simulink model "VisionModel_v8"  (Simulink 7.6)
settings: Solver=FixedStepDiscrete  StartTime=0.0  StopTime=0  RelTol=1e-3
values from neighbouring files (symbols this model uses):
  Buoy_Max_Eccentricity = 1.2    [VisionConstants.m]
  Buoy_Max_Extent = 0.9    [VisionConstants.m]
  Buoy_Min_Eccentricity = 0    [VisionConstants.m]
  Buoy_Min_Extent = 0.1    [VisionConstants.m]
  Forward_Camera_Dimensions = [160 120]    [VisionConstants.m]
  Iter_Segment_Thresh = 60    [VisionConstants.m]
  Scale_Down_B = 1    [VisionConstants.m]
  Scale_Down_G = 1    [VisionConstants.m]
  Scale_Down_H = 1    [VisionConstants.m]
  Scale_Down_R = 1    [VisionConstants.m]
  Scale_Down_S = 1    [VisionConstants.m]
  Scale_Down_V = 5    [VisionConstants.m]
  Scale_Forward_B = 0    [VisionConstants.m]
  Scale_Forward_G = 1    [VisionConstants.m]
  Scale_Forward_H = 1    [VisionConstants.m]
  Scale_Forward_R = 0    [VisionConstants.m]
  Scale_Forward_S = 1    [VisionConstants.m]
  Scale_Forward_V = 5    [VisionConstants.m]
undefined symbols (not defined in the file or in its folder): Forward_Fov, Rec, SDTV
libraries: vipconversions x8, vipgeotforms x6, viptextngfix x4, vipanalysis x2, viptransforms x2
(part 1 of 3)
settings Model: Creator=Administrator  LastModifiedBy=auvt
settings OptimizationCC: OptimizeModelRefInitCode=on
settings RTWCC: SystemTargetFile=ert.tlc  GenCodeOnly=on  TemplateMakefile=ert_default_tmf  PostCodeGenCommand=packNGo(buildInfo, {'packType' 'flat'})  Description=Real-Time Workshop Embedded Coder  GenerateReport=on  ProcessScript=ert_make_rtw_hook  IncludeHyperlinkInReport=on  LaunchReport=on  TargetLang=C++
settings CodeAppCC: IgnoreCustomStorageClasses=off
settings ERTTargetCC: MultiwordLength=2048  GenerateSampleERTMain=on  IncludeMdlTerminateFcn=off  ERTCustomFileTemplate=example_file_process.tlc  ConvertIfToSwitch=off

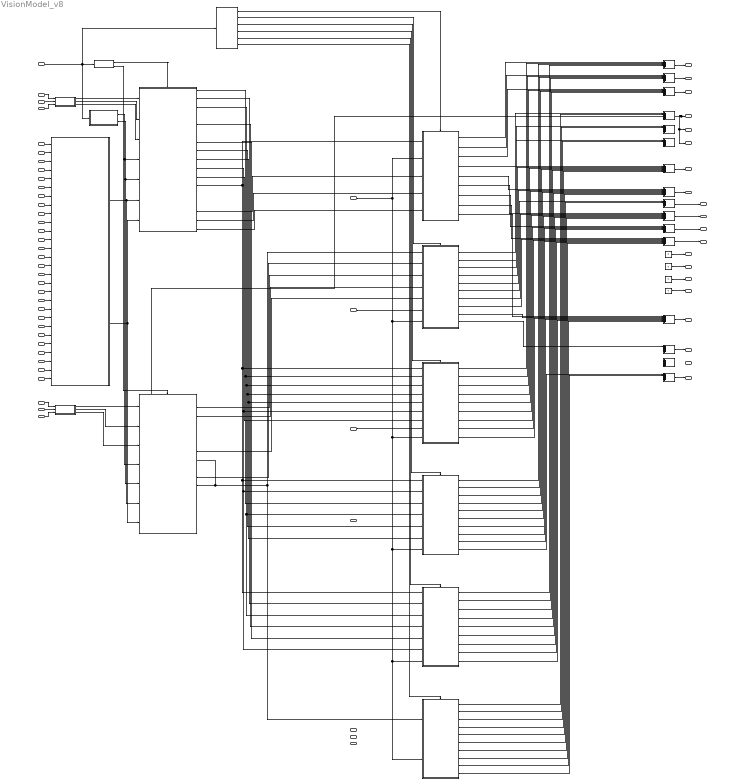
== system VisionModel_v8 ==
  note: Forward camera QImage array
  note: Down camera QImage array
  note: Forward
  note: Down
  note: Current target information
  note: Desired target information
  note: Mode and general target information
  note: Note: TargetFound, and the last three inputs to MotionController.mdl,
      | can be changed by the script, not the vision model.
  note: Path-following variables
      | DesiredPathDirection:
      | 0 = Use internal default
      | 1 = Take left path
      | 2 = Take right path
  note: Drop mechanism variables
  R_forward_in : Inport  PortDimensions=Forward_Camera_Dimensions
  G_forward_in : Inport  Port=2  PortDimensions=Forward_Camera_Dimensions
  B_forward_in : Inport  Port=3  PortDimensions=Forward_Camera_Dimensions
  R_down_in : Inport  Port=4  PortDimensions=Down_Camera_Dimensions
  G_down_in : Inport  Port=5  PortDimensions=Down_Camera_Dimensions
  B_down_in : Inport  Port=6  PortDimensions=Down_Camera_Dimensions
  ModeSelect : Inport  Port=7
  OutputImage : Inport  Port=8
  DesiredPathDirection : Inport  Port=9
  DesiredBuoyColor : Inport  Port=10
  DesiredTorpedoColor : Inport  Port=11
  ProceedToSecondTarget : Inport  Port=12
  DefaultTargetShape : Inport  Port=13
  DefaultTargetColor : Inport  Port=14
  white_al : Inport  Port=15
  white_au : Inport  Port=16
  white_bl : Inport  Port=17
  white_bu : Inport  Port=18
  black_al : Inport  Port=19
  black_au : Inport  Port=20
  black_bl : Inport  Port=21
  black_bu : Inport  Port=22
  blue_al : Inport  Port=23
  blue_au : Inport  Port=24
  blue_bl : Inport  Port=25
  blue_bu : Inport  Port=26
  red_al : Inport  Port=27
  red_au : Inport  Port=28
  red_bl : Inport  Port=29
  red_bu : Inport  Port=30
  orange_al : Inport  Port=31
  orane_au : Inport  Port=32
  orange_bl : Inport  Port=33
  orange_bu : Inport  Port=34
  yellow_al : Inport  Port=35
  yellow_au : Inport  Port=36
  yellow_bl : Inport  Port=37
  yellow_bu : Inport  Port=38
  green_al : Inport  Port=39
  green_au : Inport  Port=40
  breen_bl : Inport  Port=41
  green_bu : Inport  Port=42
  Add{,2..6,18..27} (16 alike) : Sum  Inputs=++++++
  Blob_Analysis : Subsystem  TreatAsAtomicUnit=on
  Blob_Analysis1 : Subsystem  TreatAsAtomicUnit=on
  ColorSelect : Subsystem  TreatAsAtomicUnit=on
  Constant{,1..3} (4 alike) : Constant  Value=0
  Down Filter : Subsystem
  Forward Filter : Subsystem
  If1 : If  IfExpression=u1 == 1 | u1 == 3 | u1 == 4 | u1 == 5  ElseIfExpressions=u1 == 2 | u1 == 6  ShowElse=off
  If2 : If  IfExpression=u1 == 1  ElseIfExpressions=u1 == 2, u1 == 3, u1 == 4, u1 == 5, u1 == 6  ShowElse=off
  L_detector : Subsystem  TreatAsAtomicUnit=on
  buoy_detector : Subsystem  TreatAsAtomicUnit=on
  drop_mech : Subsystem  TreatAsAtomicUnit=on
  make_color_range : Stateflow chart  TreatAsAtomicUnit=on
  path_detector : Subsystem  TreatAsAtomicUnit=on
  torpedo : Subsystem  TreatAsAtomicUnit=on
  validation_gate : Subsystem  TreatAsAtomicUnit=on
  R_forward_out : Outport  OutDataTypeStr=double
  G_forward_out : Outport  Port=2  OutDataTypeStr=double
  B_forward_out : Outport  Port=3  OutDataTypeStr=double
  R_down_out : Outport  Port=4  OutDataTypeStr=double
  G_down_out : Outport  Port=5  OutDataTypeStr=double
  B_down_out : Outport  Port=6  OutDataTypeStr=double
  TargetSelect : Outport  Port=7  OutDataTypeStr=double
  MaintainHeading : Outport  Port=8  OutDataTypeStr=double
  TargetX : Outport  Port=9  OutDataTypeStr=double
  TargetY : Outport  Port=10  OutDataTypeStr=double
  TargetZ : Outport  Port=11  OutDataTypeStr=double
  TargetYaw : Outport  Port=12  OutDataTypeStr=double
  DesiredTargetX : Outport  Port=13  OutDataTypeStr=double
  DesiredTargetY : Outport  Port=14  OutDataTypeStr=double
  DesiredTargetZ : Outport  Port=15  OutDataTypeStr=double
  DesiredTargetYaw : Outport  Port=16  OutDataTypeStr=double
  TargetDetected : Outport  Port=17  OutDataTypeStr=double
  PathState : Outport  Port=18  OutDataTypeStr=double
  BuoyColors : Outport  Port=19  OutDataTypeStr=double
  FireAuthorization : Outport  Port=20  OutDataTypeStr=double
  wires:
  G_down_in/1 -> Down Filter/2(G_in)
  R_down_in/1 -> Down Filter/1(R_in)
  B_down_in/1 -> Down Filter/3(B_in)
  If1/1 -> Blob_Analysis/Action
  If1/2 -> Blob_Analysis1/Action
  R_forward_in/1 -> Forward Filter/1(R_in)
  G_forward_in/1 -> Forward Filter/2(G_in)
  B_forward_in/1 -> Forward Filter/3(B_in)
  Blob_Analysis/12(bw_image) -> buoy_detector/1(bw_image), torpedo/1(bw_image), L_detector/1(bw_image), validation_gate/1(bw_image)
  If2/1 -> validation_gate/Action
  Add2/1 -> MaintainHeading/1
  Add3/1 -> TargetX/1
  Add4/1 -> TargetY/1
  Add5/1 -> TargetZ/1
  Add6/1 -> TargetYaw/1
  Add19/1 -> PathState/1
  Constant/1 -> DesiredTargetX/1
  Constant3/1 -> DesiredTargetYaw/1
  Constant2/1 -> DesiredTargetZ/1
  Constant1/1 -> DesiredTargetY/1
  Add21/1 -> FireAuthorization/1
  validation_gate/1(R_forward_out) -> Add22/1
  validation_gate/2(G_forward_out) -> Add23/1
  validation_gate/3(B_forward_out) -> Add24/1
  validation_gate/4(TargetSelect) -> Add/1
  validation_gate/5(MaintainHeading) -> Add2/1
  validation_gate/6(TargetY) -> Add4/1
  validation_gate/7(TargetZ) -> Add5/1
  validation_gate/8(TargetYaw) -> Add6/1
  validation_gate/9(TargetDetected) -> Add18/1
  path_detector/1(R_down_out) -> Add25/1
  path_detector/2(G_down_out) -> Add26/1
  path_detector/3(B_down_out) -> Add27/1
  path_detector/4(TargetSelect) -> Add/2
  path_detector/5(MaintainHeading) -> Add2/2
  path_detector/6(TargetX) -> Add3/1
  path_detector/7(TargetY) -> Add4/2
  path_detector/8(TargetYaw) -> Add6/2
  path_detector/9(TargetDetected) -> Add18/2
  path_detector/10(PathState) -> Add19/1
  buoy_detector/1(R_forward_out) -> Add22/2
  buoy_detector/2(G_forward_out) -> Add23/2
  buoy_detector/3(B_forward_out) -> Add24/2
  buoy_detector/4(TargetSelect) -> Add/3
  buoy_detector/5(MaintainHeading) -> Add2/3
  buoy_detector/6(TargetY) -> Add4/3
  buoy_detector/7(TargetZ) -> Add5/2
  buoy_detector/8(TargetYaw) -> Add6/3
  buoy_detector/9(TargetDetected) -> Add18/3
  ? -> Add20/1
  torpedo/1(R_forward_out) -> Add22/3
  torpedo/2(G_forward_out) -> Add23/3
  torpedo/3(B_forward_out) -> Add24/3
  torpedo/4(TargetSelect) -> Add/4
  torpedo/5(MaintainHeading) -> Add2/4
  torpedo/6(TargetY) -> Add4/4
  torpedo/7(TargetZ) -> Add5/3
  torpedo/8(TargetYaw) -> Add6/4
  torpedo/10(FireAuthorization) -> Add21/1
  torpedo/9(TargetDetected) -> Add18/4
  L_detector/1(R_forward_out) -> Add22/4
  L_detector/2(G_forward_out) -> Add23/4
  L_detector/3(B_forward_out) -> Add24/4
  L_detector/4(TargetSelect) -> Add/5
  L_detector/5(MaintainHeading) -> Add2/5
  L_detector/6(TargetY) -> Add4/5
  L_detector/7(TargetZ) -> Add5/4
  L_detector/8(TargetYaw) -> Add6/5
  L_detector/9(TargetDetected) -> Add18/5
  drop_mech/1(R_down_out) -> Add25/2
  drop_mech/2(G_down_out) -> Add26/2
  drop_mech/3(B_down_out) -> Add27/2
  drop_mech/4(TargetSelect) -> Add/6
  drop_mech/5(MaintainHeading) -> Add2/6
  drop_mech/6(TargetX) -> Add3/2
  drop_mech/7(TargetY) -> Add4/6
  drop_mech/8(TargetYaw) -> Add6/6
  drop_mech/9(TargetDetected) -> Add18/6
  drop_mech/10(FireAuthorization) -> Add21/2
  ModeSelect/1 -> If1/1, ColorSelect/1(ModeSelect), If2/1
  If2/2 -> path_detector/Action
  If2/3 -> buoy_detector/Action
  If2/4 -> torpedo/Action
  If2/5 -> L_detector/Action
  If2/6 -> drop_mech/Action
  OutputImage/1 -> validation_gate/2(output_image), buoy_detector/9(output_image), torpedo/7(output_image), drop_mech/2(output_image), L_detector/7(output_image), path_detector/7(output_image)
  DesiredBuoyColor/1 -> buoy_detector/8(DesiredBuoyColor)
  Add/1 -> TargetSelect/1
  Add18/1 -> TargetDetected/1
  Blob_Analysis/10(BlobCount) -> buoy_detector/6(blob_count), torpedo/2(blob_count), L_detector/6(blob_count)
  Blob_Analysis/1(BlobHues) -> buoy_detector/2(blob_hues), torpedo/3(blob_hues)
  Blob_Analysis/3(Centroid) -> buoy_detector/3(blob_centroids), torpedo/4(blob_centroids), L_detector/3(blob_centroid)
  Blob_Analysis/8(Eccentricity) -> buoy_detector/4(blob_eccentricity), torpedo/5(blob_eccentricity)
  Blob_Analysis/9(Extent) -> buoy_detector/5(blob_extent), torpedo/6(blob_extent)
  white_al/1 -> make_color_range/1(white_al)
  white_au/1 -> make_color_range/2(white_au)
  white_bl/1 -> make_color_range/3(white_bl)
  white_bu/1 -> make_color_range/4(white_bu)
  black_al/1 -> make_color_range/5(black_al)
  black_au/1 -> make_color_range/6(black_au)
  black_bl/1 -> make_color_range/7(black_bl)
  black_bu/1 -> make_color_range/8(black_bu)
  blue_al/1 -> make_color_range/9(blue_al)
  blue_au/1 -> make_color_range/10(blue_au)
  blue_bl/1 -> make_color_range/11(blue_bl)
  blue_bu/1 -> make_color_range/12(blue_bu)
  red_al/1 -> make_color_range/13(red_al)
  red_au/1 -> make_color_range/14(red_au)
  red_bl/1 -> make_color_range/15(red_bl)
  red_bu/1 -> make_color_range/16(red_bu)
  orange_al/1 -> make_color_range/17(orange_al)
  orane_au/1 -> make_color_range/18(orange_au)
  orange_bl/1 -> make_color_range/19(orange_bl)
  orange_bu/1 -> make_color_range/20(orange_bu)
  yellow_al/1 -> make_color_range/21(yellow_al)
  yellow_au/1 -> make_color_range/22(yellow_au)
  yellow_bl/1 -> make_color_range/23(yellow_bl)
  yellow_bu/1 -> make_color_range/24(yellow_bu)
  green_al/1 -> make_color_range/25(green_al)
  green_au/1 -> make_color_range/26(green_au)
  breen_bl/1 -> make_color_range/27(green_bl)
  green_bu/1 -> make_color_range/28(green_bu)
  make_color_range/1(a_range) -> Blob_Analysis/6(a_range), Blob_Analysis1/6(a_range)
  Forward Filter/1(R_out) -> Blob_Analysis/1(R_in)
  Forward Filter/2(G_out) -> Blob_Analysis/2(G_in)
  Forward Filter/3(B_out) -> Blob_Analysis/3(B_in)
  Blob_Analysis/2(Area) -> L_detector/2(blob_area)
  Blob_Analysis/5(MajorAxis) -> L_detector/4(blob_major_axis)
  Blob_Analysis/7(Orientation) -> L_detector/5(blob_orientation)
  ColorSelect/1(ColorFilter) -> Blob_Analysis/4(ColorFilter), Blob_Analysis1/4(ColorFilter)
  ColorSelect/2(OutputSegmentedImage) -> Blob_Analysis/5(OutputSegmentedImage), Blob_Analysis1/5(OutputSegmentedImage)
  Down Filter/1(R_out) -> Blob_Analysis1/1(R_in)
  Down Filter/2(G_out) -> Blob_Analysis1/2(G_in)
  Down Filter/3(B_out) -> Blob_Analysis1/3(B_in)
  make_color_range/2(b_range) -> Blob_Analysis/7(b_range), Blob_Analysis1/7(b_range)
  Blob_Analysis1/11(bw_image) -> path_detector/1(bw_image), drop_mech/1(bw_image), R_down_out/1, G_down_out/1, B_down_out/1
  Blob_Analysis1/10(BlobCount) -> path_detector/2(blob_count)
  Blob_Analysis1/2(Area) -> path_detector/3(blob_area)
  Blob_Analysis1/3(Centroid) -> path_detector/4(blob_centroids)
  Blob_Analysis1/7(Orientation) -> path_detector/5(blob_orientation)
  DesiredPathDirection/1 -> path_detector/6(DesiredPathDirection)
  Add22/1 -> R_forward_out/1
  Add23/1 -> G_forward_out/1
  Add24/1 -> B_forward_out/1
  Blob_Analysis/15(R_out) -> validation_gate/3(R_in)
  Blob_Analysis/16(G_out) -> validation_gate/4(G_in)
  Blob_Analysis/17(B_out) -> validation_gate/5(B_in)
  ? -> BuoyColors/1
  Blob_Analysis/11(BlobColor) -> buoy_detector/7(blob_colors)

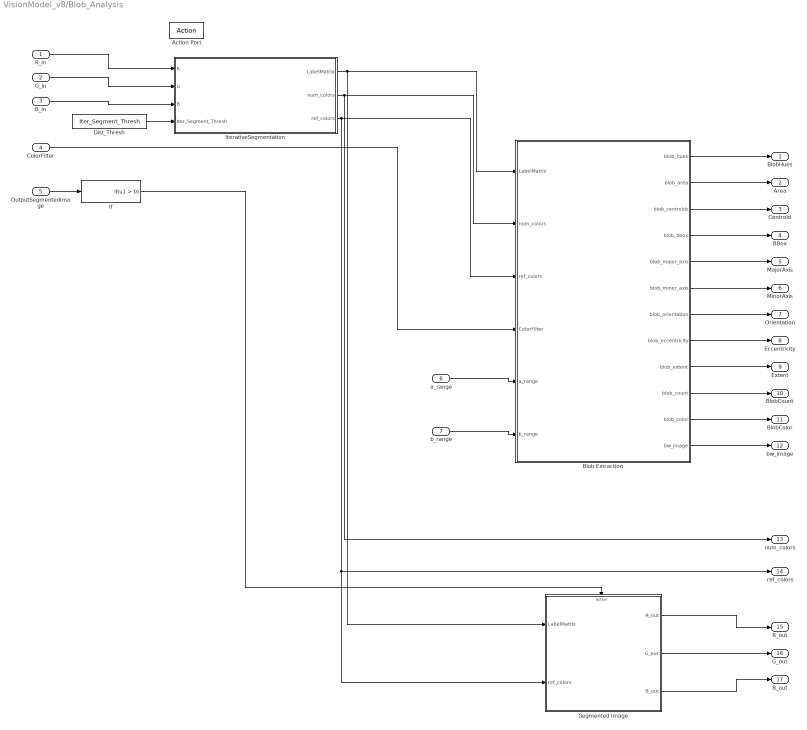
== system VisionModel_v8/Blob_Analysis ==
  R_in : Inport
  G_in : Inport  Port=2
  B_in : Inport  Port=3
  ColorFilter : Inport  Port=4
  OutputSegmentedImage : Inport  Port=5
  a_range : Inport  Port=6
  b_range : Inport  Port=7
  Action Port : ActionPort  ActionType=then
  Blob Extraction : Stateflow chart  TreatAsAtomicUnit=on
  Dist_Thresh : Constant  Value=Iter_Segment_Thresh  SampleTime=-1
  If : If  ShowElse=off
  IterativeSegmentation : Subsystem
      settings: UndoDeleteFcn=Stateflow.SLINSF.SimulinkMan.restorePreDeleteFcn  PreDeleteFcn=Stateflow.SLINSF.SimulinkMan.removePreDeleteFcn
  Segmented Image : Subsystem  TreatAsAtomicUnit=on
  BlobHues : Outport
  Area : Outport  Port=2
  Centroid : Outport  Port=3
  BBox : Outport  Port=4
  MajorAxis : Outport  Port=5
  MinorAxis : Outport  Port=6
  Orientation : Outport  Port=7
  Eccentricity : Outport  Port=8
  Extent : Outport  Port=9
  BlobCount : Outport  Port=10
  BlobColor : Outport  Port=11
  bw_image : Outport  Port=12
  num_colors : Outport  Port=13
  ref_colors : Outport  Port=14
  R_out : Outport  Port=15
  G_out : Outport  Port=16
  B_out : Outport  Port=17
  wires:
  Blob Extraction/12(bw_image) -> bw_image/1
  Blob Extraction/10(blob_count) -> BlobCount/1
  Blob Extraction/9(blob_extent) -> Extent/1
  Blob Extraction/8(blob_eccentricity) -> Eccentricity/1
  Blob Extraction/7(blob_orientation) -> Orientation/1
  Blob Extraction/6(blob_minor_axis) -> MinorAxis/1
  Blob Extraction/5(blob_major_axis) -> MajorAxis/1
  Blob Extraction/4(blob_bbox) -> BBox/1
  Blob Extraction/3(blob_centroids) -> Centroid/1
  Blob Extraction/2(blob_area) -> Area/1
  Blob Extraction/1(blob_hues) -> BlobHues/1
  ColorFilter/1 -> Blob Extraction/4(ColorFilter)
  a_range/1 -> Blob Extraction/5(a_range)
  b_range/1 -> Blob Extraction/6(b_range)
  IterativeSegmentation/1(LabelMatrix) -> Blob Extraction/1(LabelMatrix), Segmented Image/1(LabelMatrix)
  IterativeSegmentation/2(num_colors) -> Blob Extraction/2(num_colors), num_colors/1
  IterativeSegmentation/3(ref_colors) -> Blob Extraction/3(ref_colors), Segmented Image/2(ref_colors), ref_colors/1
  Dist_Thresh/1 -> IterativeSegmentation/4(Iter_Segment_Thresh)
  R_in/1 -> IterativeSegmentation/1(R)
  G_in/1 -> IterativeSegmentation/2(G)
  B_in/1 -> IterativeSegmentation/3(B)
  If/1 -> Segmented Image/Action
  OutputSegmentedImage/1 -> If/1
  Segmented Image/1(R_out) -> R_out/1
  Segmented Image/2(G_out) -> G_out/1
  Segmented Image/3(B_out) -> B_out/1
  Blob Extraction/11(blob_color) -> BlobColor/1

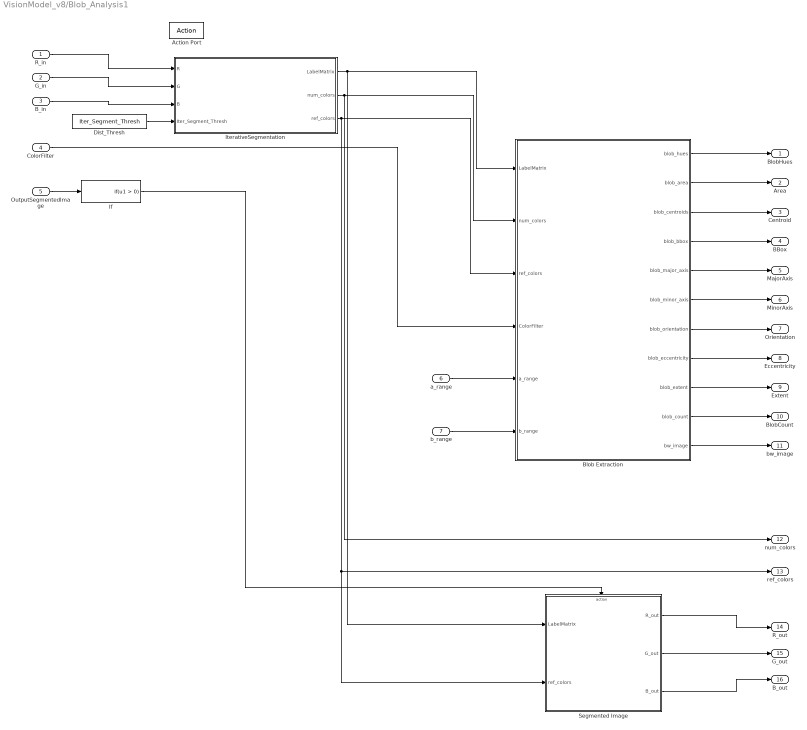
== system VisionModel_v8/Blob_Analysis1 ==
  R_in : Inport
  G_in : Inport  Port=2
  B_in : Inport  Port=3
  ColorFilter : Inport  Port=4
  OutputSegmentedImage : Inport  Port=5
  a_range : Inport  Port=6
  b_range : Inport  Port=7
  Action Port : ActionPort  ActionType=elseif
  Blob Extraction : Stateflow chart  TreatAsAtomicUnit=on
  Dist_Thresh : Constant  Value=Iter_Segment_Thresh  SampleTime=-1
  If : If  ShowElse=off
  IterativeSegmentation : Subsystem
      settings: UndoDeleteFcn=Stateflow.SLINSF.SimulinkMan.restorePreDeleteFcn  PreDeleteFcn=Stateflow.SLINSF.SimulinkMan.removePreDeleteFcn
  Segmented Image : Subsystem  TreatAsAtomicUnit=on
  BlobHues : Outport
  Area : Outport  Port=2
  Centroid : Outport  Port=3
  BBox : Outport  Port=4
  MajorAxis : Outport  Port=5
  MinorAxis : Outport  Port=6
  Orientation : Outport  Port=7
  Eccentricity : Outport  Port=8
  Extent : Outport  Port=9
  BlobCount : Outport  Port=10
  bw_image : Outport  Port=11
  num_colors : Outport  Port=12
  ref_colors : Outport  Port=13
  R_out : Outport  Port=14
  G_out : Outport  Port=15
  B_out : Outport  Port=16
  wires:
  Segmented Image/3(B_out) -> B_out/1
  Segmented Image/2(G_out) -> G_out/1
  Segmented Image/1(R_out) -> R_out/1
  OutputSegmentedImage/1 -> If/1
  If/1 -> Segmented Image/Action
  B_in/1 -> IterativeSegmentation/3(B)
  G_in/1 -> IterativeSegmentation/2(G)
  R_in/1 -> IterativeSegmentation/1(R)
  Dist_Thresh/1 -> IterativeSegmentation/4(Iter_Segment_Thresh)
  IterativeSegmentation/3(ref_colors) -> ref_colors/1, Segmented Image/2(ref_colors), Blob Extraction/3(ref_colors)
  IterativeSegmentation/2(num_colors) -> num_colors/1, Blob Extraction/2(num_colors)
  IterativeSegmentation/1(LabelMatrix) -> Segmented Image/1(LabelMatrix), Blob Extraction/1(LabelMatrix)
  b_range/1 -> Blob Extraction/6(b_range)
  a_range/1 -> Blob Extraction/5(a_range)
  ColorFilter/1 -> Blob Extraction/4(ColorFilter)
  Blob Extraction/1(blob_hues) -> BlobHues/1
  Blob Extraction/2(blob_area) -> Area/1
  Blob Extraction/3(blob_centroids) -> Centroid/1
  Blob Extraction/4(blob_bbox) -> BBox/1
  Blob Extraction/5(blob_major_axis) -> MajorAxis/1
  Blob Extraction/6(blob_minor_axis) -> MinorAxis/1
  Blob Extraction/7(blob_orientation) -> Orientation/1
  Blob Extraction/8(blob_eccentricity) -> Eccentricity/1
  Blob Extraction/9(blob_extent) -> Extent/1
  Blob Extraction/10(blob_count) -> BlobCount/1
  Blob Extraction/11(bw_image) -> bw_image/1

== system VisionModel_v8/ColorSelect ==
  ModeSelect : Inport
  Add1 : Sum  Inputs=++++++
  Add22 : Sum  Inputs=++++++
  If3 : If  IfExpression=u1 == 1  ElseIfExpressions=u1 == 2, u1 == 3, u1 == 4, u1 == 5, u1 == 6  ShowElse=off
  L_detector : Subsystem  TreatAsAtomicUnit=on
  buoy_detector : Subsystem  TreatAsAtomicUnit=on
  drop_mech : Subsystem  TreatAsAtomicUnit=on
  path_detector : Subsystem  TreatAsAtomicUnit=on
  torpedo : Subsystem  TreatAsAtomicUnit=on
  validation_gate : Subsystem  TreatAsAtomicUnit=on
  ColorFilter : Outport  OutDataTypeStr=double
  OutputSegmentedImage : Outport  Port=2  OutDataTypeStr=double
  wires:
  ModeSelect/1 -> If3/1
  If3/1 -> validation_gate/Action
  Add22/1 -> ColorFilter/1
  If3/2 -> path_detector/Action
  If3/3 -> buoy_detector/Action
  If3/4 -> torpedo/Action
  If3/5 -> L_detector/Action
  If3/6 -> drop_mech/Action
  Add1/1 -> OutputSegmentedImage/1
  validation_gate/1(ColorFilter) -> Add22/1
  validation_gate/2(OutputSegmentedImage) -> Add1/1
  path_detector/1(ColorFilter) -> Add22/2
  path_detector/2(OutputSegmentedImage) -> Add1/2
  buoy_detector/1(ColorFilter) -> Add22/3
  buoy_detector/2(OutputSegmentedImage) -> Add1/3
  torpedo/1(ColorFilter) -> Add22/4
  torpedo/2(OutputSegmentedImage) -> Add1/4
  L_detector/1(ColorFilter) -> Add22/5
  L_detector/2(OutputSegmentedImage) -> Add1/5
  drop_mech/1(ColorFilter) -> Add22/6
  drop_mech/2(OutputSegmentedImage) -> Add1/6

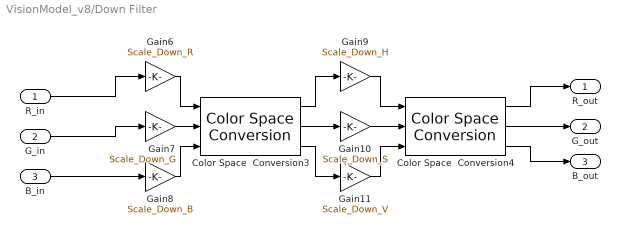
== system VisionModel_v8/Down Filter ==
  R_in : Inport  PortDimensions=Down_Camera_Dimensions
  G_in : Inport  Port=2  PortDimensions=Down_Camera_Dimensions
  B_in : Inport  Port=3  PortDimensions=Down_Camera_Dimensions
  Color Space  Conversion3 : vipconversions/Color Space  Conversion  conversion=Obsolete  conversionActive=R'G'B' to HSV  wp_str=D50  rec=Rec. 601 (SDTV)  sys=1125/60/2:1  imagePorts=Separate color signals
  Color Space  Conversion4 : vipconversions/Color Space  Conversion  conversion=Obsolete  conversionActive=HSV to R'G'B'  wp_str=D50  rec=Rec. 601 (SDTV)  sys=1125/60/2:1  imagePorts=Separate color signals
  Gain10 : Gain  Gain=Scale_Down_S
  Gain11 : Gain  Gain=Scale_Down_V
  Gain6 : Gain  Gain=Scale_Down_R
  Gain7 : Gain  Gain=Scale_Down_G
  Gain8 : Gain  Gain=Scale_Down_B
  Gain9 : Gain  Gain=Scale_Down_H
  R_out : Outport  OutDataTypeStr=double
  G_out : Outport  Port=2  OutDataTypeStr=double
  B_out : Outport  Port=3  OutDataTypeStr=double
  wires:
  Gain6/1 -> Color Space  Conversion3/1
  Gain7/1 -> Color Space  Conversion3/2
  Gain8/1 -> Color Space  Conversion3/3
  Color Space  Conversion3/1 -> Gain9/1
  Color Space  Conversion3/2 -> Gain10/1
  Color Space  Conversion3/3 -> Gain11/1
  Gain9/1 -> Color Space  Conversion4/1
  Gain10/1 -> Color Space  Conversion4/2
  Gain11/1 -> Color Space  Conversion4/3
  R_in/1 -> Gain6/1
  G_in/1 -> Gain7/1
  B_in/1 -> Gain8/1
  Color Space  Conversion4/1 -> R_out/1
  Color Space  Conversion4/2 -> G_out/1
  Color Space  Conversion4/3 -> B_out/1

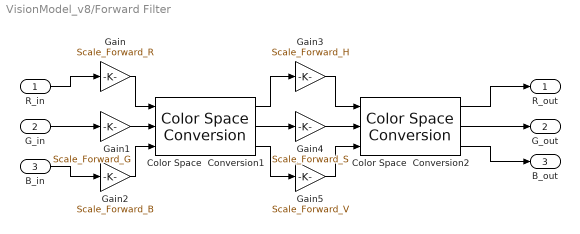
== system VisionModel_v8/Forward Filter ==
  R_in : Inport  PortDimensions=Forward_Camera_Dimensions
  G_in : Inport  Port=2  PortDimensions=Forward_Camera_Dimensions
  B_in : Inport  Port=3  PortDimensions=Forward_Camera_Dimensions
  Color Space  Conversion1 : vipconversions/Color Space  Conversion  conversion=Obsolete  conversionActive=R'G'B' to HSV  wp_str=D50  rec=Rec. 601 (SDTV)  sys=1125/60/2:1  imagePorts=Separate color signals
  Color Space  Conversion2 : vipconversions/Color Space  Conversion  conversion=Obsolete  conversionActive=HSV to R'G'B'  wp_str=D50  rec=Rec. 601 (SDTV)  sys=1125/60/2:1  imagePorts=Separate color signals
  Gain : Gain  Gain=Scale_Forward_R
  Gain1 : Gain  Gain=Scale_Forward_G
  Gain2 : Gain  Gain=Scale_Forward_B
  Gain3 : Gain  Gain=Scale_Forward_H
  Gain4 : Gain  Gain=Scale_Forward_S
  Gain5 : Gain  Gain=Scale_Forward_V
  R_out : Outport  OutDataTypeStr=double
  G_out : Outport  Port=2  OutDataTypeStr=double
  B_out : Outport  Port=3  OutDataTypeStr=double
  wires:
  R_in/1 -> Gain/1
  G_in/1 -> Gain1/1
  B_in/1 -> Gain2/1
  Gain/1 -> Color Space  Conversion1/1
  Gain1/1 -> Color Space  Conversion1/2
  Gain2/1 -> Color Space  Conversion1/3
  Color Space  Conversion1/1 -> Gain3/1
  Color Space  Conversion1/2 -> Gain4/1
  Color Space  Conversion1/3 -> Gain5/1
  Gain3/1 -> Color Space  Conversion2/1
  Gain4/1 -> Color Space  Conversion2/2
  Gain5/1 -> Color Space  Conversion2/3
  Color Space  Conversion2/1 -> R_out/1
  Color Space  Conversion2/2 -> G_out/1
  Color Space  Conversion2/3 -> B_out/1

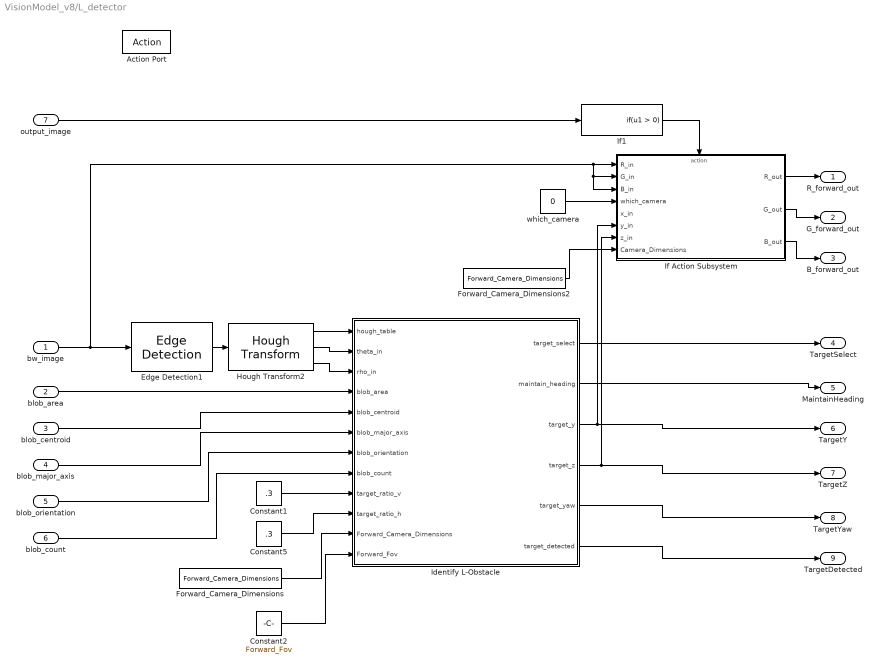
== system VisionModel_v8/L_detector ==
  bw_image : Inport
  blob_area : Inport  Port=2
  blob_centroid : Inport  Port=3
  blob_major_axis : Inport  Port=4
  blob_orientation : Inport  Port=5
  blob_count : Inport  Port=6
  output_image : Inport  Port=7
  Action Port : ActionPort  ActionType=elseif
  Constant1 : Constant  Value=.3  SampleTime=-1
  Constant2 : Constant  Value=Forward_Fov  SampleTime=-1
  Constant5 : Constant  Value=.3  SampleTime=-1
  Edge Detection1 : vipanalysis/Edge Detection  DialogController=vipDDGCreate  DialogControllerArgs=DataTag6  method=Sobel  outputType=Binary image  userDefinedThreshold=off  thresholdSource=Specify via dialog  threshold=20  thresholdTuning=3  edgeThinning=on  threshold_canny=[0.25 0.60]  autoPercent=70  sigma=1  roundingMode=Floor  overflowMode=off
  Forward_Camera_Dimensions : Constant  Value=Forward_Camera_Dimensions  SampleTime=-1
  Forward_Camera_Dimensions2 : Constant  Value=Forward_Camera_Dimensions  SampleTime=-1
  Hough Transform2 : viptransforms/Hough Transform  DialogController=vipDDGCreate  DialogControllerArgs=DataTag7  theta_res=pi/180  rho_res=1  out_theta_rho=on  outdtmode=double  firstCoeffMode=Binary point scaling  firstCoeffWordLength=16  firstCoeffFracLength=14  secondCoeffMode=Binary point scaling  secondCoeffWordLength=32  secondCoeffFracLength=16  outputMode=Binary point scaling  outputWordLength=16  outputFracLength=0  accumMode=Binary point scaling  accumWordLength=32  accumFracLength=20  prodOutputMode=Binary point scaling  prodOutputWordLength=32  prodOutputFracLength=20  memoryMode=Binary point scaling  memoryWordLength=32  memoryFracLength=16  roundingMode=Nearest  overflowMode=on
  Identify L-Obstacle : Stateflow chart  TreatAsAtomicUnit=on  SystemSampleTime=[1/30 0]
  If Action Subsystem : Subsystem  TreatAsAtomicUnit=on
  If1 : If  ShowElse=off
  which_camera : Constant  Value=0  SampleTime=-1
  R_forward_out : Outport  OutDataTypeStr=double
  G_forward_out : Outport  Port=2  OutDataTypeStr=double
  B_forward_out : Outport  Port=3  OutDataTypeStr=double
  TargetSelect : Outport  Port=4  OutDataTypeStr=double
  MaintainHeading : Outport  Port=5  OutDataTypeStr=double
  TargetY : Outport  Port=6  OutDataTypeStr=double
  TargetZ : Outport  Port=7  OutDataTypeStr=double
  TargetYaw : Outport  Port=8  OutDataTypeStr=double
  TargetDetected : Outport  Port=9  OutDataTypeStr=double
  wires:
  Identify L-Obstacle/1(target_select) -> TargetSelect/1
  Identify L-Obstacle/2(maintain_heading) -> MaintainHeading/1
  Identify L-Obstacle/3(target_y) -> TargetY/1, If Action Subsystem/6(y_in)
  Identify L-Obstacle/4(target_z) -> TargetZ/1, If Action Subsystem/7(z_in)
  Identify L-Obstacle/5(target_yaw) -> TargetYaw/1
  Identify L-Obstacle/6(target_detected) -> TargetDetected/1
  Edge Detection1/1 -> Hough Transform2/1
  Hough Transform2/1 -> Identify L-Obstacle/1(hough_table)
  Hough Transform2/2 -> Identify L-Obstacle/2(theta_in)
  Hough Transform2/3 -> Identify L-Obstacle/3(rho_in)
  bw_image/1 -> Edge Detection1/1, If Action Subsystem/1(R_in), If Action Subsystem/2(G_in), If Action Subsystem/3(B_in)
  If1/1 -> If Action Subsystem/Action
  which_camera/1 -> If Action Subsystem/4(which_camera)
  Forward_Camera_Dimensions2/1 -> If Action Subsystem/8(Camera_Dimensions)
  If Action Subsystem/1(R_out) -> R_forward_out/1
  If Action Subsystem/2(G_out) -> G_forward_out/1
  If Action Subsystem/3(B_out) -> B_forward_out/1
  output_image/1 -> If1/1
  blob_area/1 -> Identify L-Obstacle/4(blob_area)
  blob_centroid/1 -> Identify L-Obstacle/5(blob_centroid)
  blob_major_axis/1 -> Identify L-Obstacle/6(blob_major_axis)
  blob_orientation/1 -> Identify L-Obstacle/7(blob_orientation)
  blob_count/1 -> Identify L-Obstacle/8(blob_count)
  Constant1/1 -> Identify L-Obstacle/9(target_ratio_v)
  Constant5/1 -> Identify L-Obstacle/10(target_ratio_h)
  Forward_Camera_Dimensions/1 -> Identify L-Obstacle/11(Forward_Camera_Dimensions)
  Constant2/1 -> Identify L-Obstacle/12(Forward_Fov)

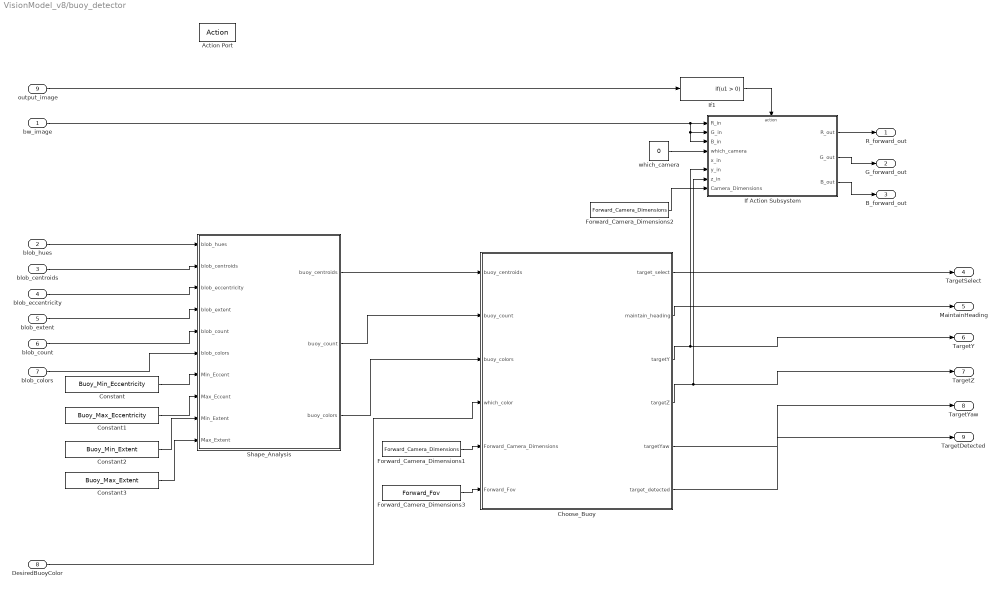
== system VisionModel_v8/buoy_detector ==
  bw_image : Inport
  blob_hues : Inport  Port=2
  blob_centroids : Inport  Port=3
  blob_eccentricity : Inport  Port=4
  blob_extent : Inport  Port=5
  blob_count : Inport  Port=6
  blob_colors : Inport  Port=7
  DesiredBuoyColor : Inport  Port=8
  output_image : Inport  Port=9
  Action Port : ActionPort  ActionType=elseif
  Choose_Buoy : Stateflow chart  TreatAsAtomicUnit=on
  Constant : Constant  Value=Buoy_Min_Eccentricity  SampleTime=-1
  Constant1 : Constant  Value=Buoy_Max_Eccentricity  SampleTime=-1
  Constant2 : Constant  Value=Buoy_Min_Extent  SampleTime=-1
  Constant3 : Constant  Value=Buoy_Max_Extent  SampleTime=-1
  Forward_Camera_Dimensions1 : Constant  Value=Forward_Camera_Dimensions  SampleTime=-1
  Forward_Camera_Dimensions2 : Constant  Value=Forward_Camera_Dimensions  SampleTime=-1
  Forward_Camera_Dimensions3 : Constant  Value=Forward_Fov  SampleTime=-1
  If Action Subsystem : Subsystem  TreatAsAtomicUnit=on
  If1 : If  ShowElse=off
  Shape_Analysis : Stateflow chart  TreatAsAtomicUnit=on
  which_camera : Constant  Value=0  SampleTime=-1
  R_forward_out : Outport  OutDataTypeStr=double
  G_forward_out : Outport  Port=2  OutDataTypeStr=double
  B_forward_out : Outport  Port=3  OutDataTypeStr=double
  TargetSelect : Outport  Port=4  OutDataTypeStr=double
  MaintainHeading : Outport  Port=5  OutDataTypeStr=double
  TargetY : Outport  Port=6  OutDataTypeStr=double
  TargetZ : Outport  Port=7  OutDataTypeStr=double
  TargetYaw : Outport  Port=8  OutDataTypeStr=double
  TargetDetected : Outport  Port=9  OutDataTypeStr=double
  wires:
  Choose_Buoy/1(target_select) -> TargetSelect/1
  Choose_Buoy/2(maintain_heading) -> MaintainHeading/1
  Choose_Buoy/3(targetY) -> TargetY/1, If Action Subsystem/6(y_in)
  Choose_Buoy/4(targetZ) -> TargetZ/1, If Action Subsystem/7(z_in)
  Choose_Buoy/5(targetYaw) -> TargetYaw/1
  Choose_Buoy/6(target_detected) -> TargetDetected/1
  Forward_Camera_Dimensions1/1 -> Choose_Buoy/5(Forward_Camera_Dimensions)
  If1/1 -> If Action Subsystem/Action
  which_camera/1 -> If Action Subsystem/4(which_camera)
  Forward_Camera_Dimensions2/1 -> If Action Subsystem/8(Camera_Dimensions)
  output_image/1 -> If1/1
  blob_hues/1 -> Shape_Analysis/1(blob_hues)
  blob_centroids/1 -> Shape_Analysis/2(blob_centroids)
  blob_eccentricity/1 -> Shape_Analysis/3(blob_eccentricity)
  blob_extent/1 -> Shape_Analysis/4(blob_extent)
  blob_count/1 -> Shape_Analysis/5(blob_count)
  Constant/1 -> Shape_Analysis/7(Min_Eccent)
  Constant1/1 -> Shape_Analysis/8(Max_Eccent)
  Constant2/1 -> Shape_Analysis/9(Min_Extent)
  Constant3/1 -> Shape_Analysis/10(Max_Extent)
  blob_colors/1 -> Shape_Analysis/6(blob_colors)
  Forward_Camera_Dimensions3/1 -> Choose_Buoy/6(Forward_Fov)
  Shape_Analysis/1(buoy_centroids) -> Choose_Buoy/1(buoy_centroids)
  Shape_Analysis/2(buoy_count) -> Choose_Buoy/2(buoy_count)
  Shape_Analysis/3(buoy_colors) -> Choose_Buoy/3(buoy_colors)
  DesiredBuoyColor/1 -> Choose_Buoy/4(which_color)
  If Action Subsystem/1(R_out) -> R_forward_out/1
  If Action Subsystem/2(G_out) -> G_forward_out/1
  If Action Subsystem/3(B_out) -> B_forward_out/1
  bw_image/1 -> If Action Subsystem/1(R_in), If Action Subsystem/2(G_in), If Action Subsystem/3(B_in)

== system VisionModel_v8/drop_mech ==
  bw_image : Inport
  output_image : Inport  Port=2
  Action Port : ActionPort  ActionType=elseif
  R_down_out : Outport  OutDataTypeStr=double
  G_down_out : Outport  Port=2  OutDataTypeStr=double
  B_down_out : Outport  Port=3  OutDataTypeStr=double
  TargetSelect : Outport  Port=4  OutDataTypeStr=double
  MaintainHeading : Outport  Port=5  OutDataTypeStr=double
  TargetX : Outport  Port=6  OutDataTypeStr=double
  TargetY : Outport  Port=7  OutDataTypeStr=double
  TargetYaw : Outport  Port=8  OutDataTypeStr=double
  TargetDetected : Outport  Port=9  OutDataTypeStr=double
  FireAuthorization : Outport  Port=10  OutDataTypeStr=double

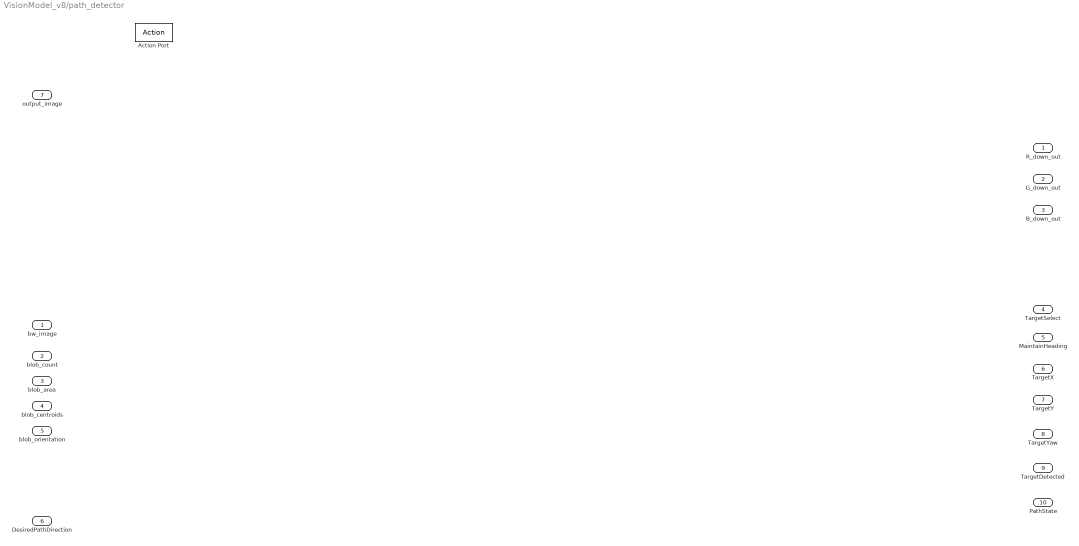
== system VisionModel_v8/path_detector ==
  bw_image : Inport
  blob_count : Inport  Port=2
  blob_area : Inport  Port=3
  blob_centroids : Inport  Port=4
  blob_orientation : Inport  Port=5
  DesiredPathDirection : Inport  Port=6
  output_image : Inport  Port=7
  Action Port : ActionPort  ActionType=elseif
  R_down_out : Outport  OutDataTypeStr=double
  G_down_out : Outport  Port=2  OutDataTypeStr=double
  B_down_out : Outport  Port=3  OutDataTypeStr=double
  TargetSelect : Outport  Port=4  OutDataTypeStr=double
  MaintainHeading : Outport  Port=5  OutDataTypeStr=double
  TargetX : Outport  Port=6  OutDataTypeStr=double
  TargetY : Outport  Port=7  OutDataTypeStr=double
  TargetYaw : Outport  Port=8  OutDataTypeStr=double
  TargetDetected : Outport  Port=9  OutDataTypeStr=double
  PathState : Outport  Port=10  OutDataTypeStr=double

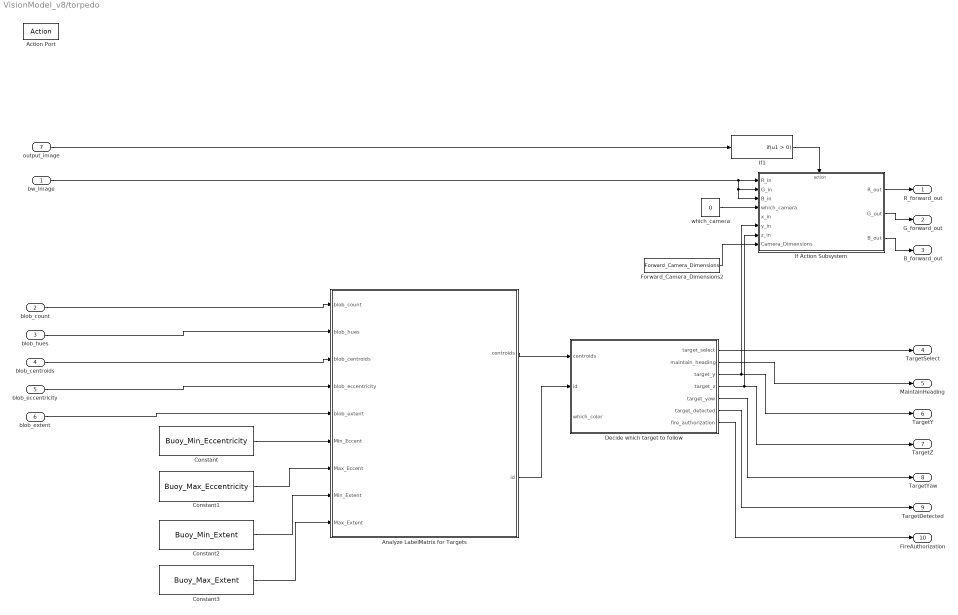
== system VisionModel_v8/torpedo ==
  bw_image : Inport
  blob_count : Inport  Port=2
  blob_hues : Inport  Port=3
  blob_centroids : Inport  Port=4
  blob_eccentricity : Inport  Port=5
  blob_extent : Inport  Port=6
  output_image : Inport  Port=7
  Action Port : ActionPort  ActionType=elseif
  Analyze LabelMatrix for Targets : Stateflow chart  TreatAsAtomicUnit=on
  Constant : Constant  Value=Buoy_Min_Eccentricity  SampleTime=-1
  Constant1 : Constant  Value=Buoy_Max_Eccentricity  SampleTime=-1
  Constant2 : Constant  Value=Buoy_Min_Extent  SampleTime=-1
  Constant3 : Constant  Value=Buoy_Max_Extent  SampleTime=-1
  Decide which target to follow : Stateflow chart  TreatAsAtomicUnit=on
  Forward_Camera_Dimensions2 : Constant  Value=Forward_Camera_Dimensions  SampleTime=-1
  If Action Subsystem : Subsystem  TreatAsAtomicUnit=on
  If1 : If  ShowElse=off
  which_camera : Constant  Value=0  SampleTime=-1
  R_forward_out : Outport  OutDataTypeStr=double
  G_forward_out : Outport  Port=2  OutDataTypeStr=double
  B_forward_out : Outport  Port=3  OutDataTypeStr=double
  TargetSelect : Outport  Port=4  OutDataTypeStr=double
  MaintainHeading : Outport  Port=5  OutDataTypeStr=double
  TargetY : Outport  Port=6  OutDataTypeStr=double
  TargetZ : Outport  Port=7  OutDataTypeStr=double
  TargetYaw : Outport  Port=8  OutDataTypeStr=double
  TargetDetected : Outport  Port=9  OutDataTypeStr=double
  FireAuthorization : Outport  Port=10  OutDataTypeStr=double
  wires:
  Decide which target to follow/3(target_y) -> TargetY/1, If Action Subsystem/6(y_in)
  Decide which target to follow/4(target_z) -> TargetZ/1, If Action Subsystem/7(z_in)
  Decide which target to follow/5(target_yaw) -> TargetYaw/1
  Decide which target to follow/6(target_detected) -> TargetDetected/1
  Decide which target to follow/7(fire_authorization) -> FireAuthorization/1
  Analyze LabelMatrix for Targets/1(centroids) -> Decide which target to follow/1(centroids)
  Analyze LabelMatrix for Targets/2(id) -> Decide which target to follow/2(id)
  Constant/1 -> Analyze LabelMatrix for Targets/6(Min_Eccent)
  Constant1/1 -> Analyze LabelMatrix for Targets/7(Max_Eccent)
  Constant2/1 -> Analyze LabelMatrix for Targets/8(Min_Extent)
  Constant3/1 -> Analyze LabelMatrix for Targets/9(Max_Extent)
  blob_count/1 -> Analyze LabelMatrix for Targets/1(blob_count)
  blob_hues/1 -> Analyze LabelMatrix for Targets/2(blob_hues)
  blob_centroids/1 -> Analyze LabelMatrix for Targets/3(blob_centroids)
  blob_eccentricity/1 -> Analyze LabelMatrix for Targets/4(blob_eccentricity)
  blob_extent/1 -> Analyze LabelMatrix for Targets/5(blob_extent)
  If1/1 -> If Action Subsystem/Action
  which_camera/1 -> If Action Subsystem/4(which_camera)
  Forward_Camera_Dimensions2/1 -> If Action Subsystem/8(Camera_Dimensions)
  If Action Subsystem/1(R_out) -> R_forward_out/1
  If Action Subsystem/2(G_out) -> G_forward_out/1
  If Action Subsystem/3(B_out) -> B_forward_out/1
  bw_image/1 -> If Action Subsystem/1(R_in), If Action Subsystem/2(G_in), If Action Subsystem/3(B_in)
  output_image/1 -> If1/1
  Decide which target to follow/2(maintain_heading) -> MaintainHeading/1
  Decide which target to follow/1(target_select) -> TargetSelect/1

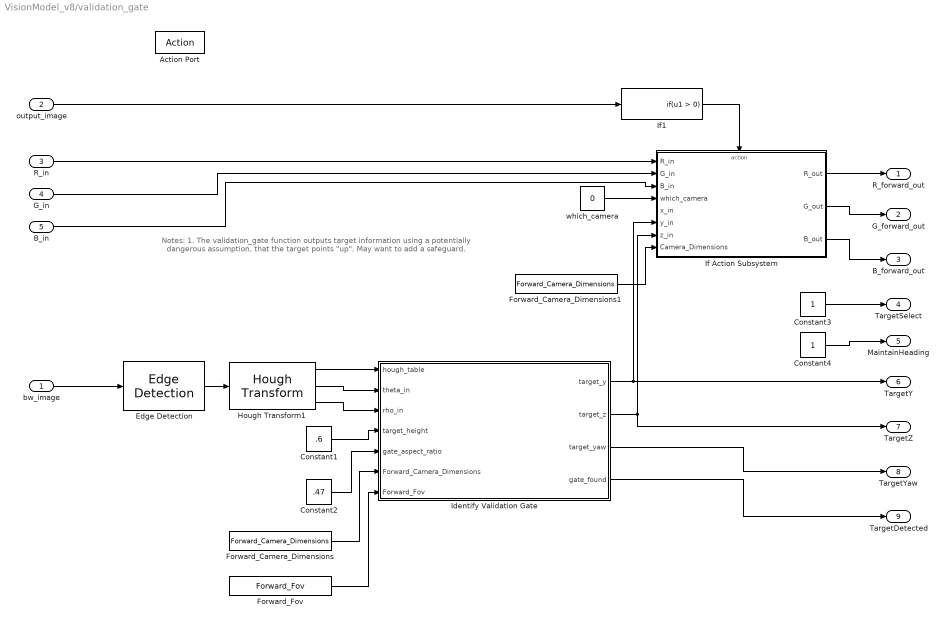
== system VisionModel_v8/validation_gate ==
  note: Notes:
      | 1. The validation_gate function outputs target
      | information using a potentially dangerous
      | assumption, that the target points "up". May
      | want to add a safeguard.
  bw_image : Inport  PortDimensions=Forward_Camera_Dimensions
  output_image : Inport  Port=2
  R_in : Inport  Port=3
  G_in : Inport  Port=4
  B_in : Inport  Port=5
  Action Port : ActionPort  ActionType=then
  Constant1 : Constant  Value=.6  SampleTime=-1
  Constant2 : Constant  Value=.47  SampleTime=-1
  Constant3 : Constant  SampleTime=-1
  Constant4 : Constant  SampleTime=-1
  Edge Detection : vipanalysis/Edge Detection  DialogController=vipDDGCreate  DialogControllerArgs=DataTag11  method=Sobel  outputType=Binary image  userDefinedThreshold=off  thresholdSource=Specify via dialog  threshold=0  thresholdTuning=3  edgeThinning=on  threshold_canny=[0.25 0.60]  autoPercent=70  sigma=1  roundingMode=Floor  overflowMode=off
  Forward_Camera_Dimensions : Constant  Value=Forward_Camera_Dimensions  SampleTime=-1
  Forward_Camera_Dimensions1 : Constant  Value=Forward_Camera_Dimensions  SampleTime=-1
  Forward_Fov : Constant  Value=Forward_Fov  SampleTime=-1
  Hough Transform1 : viptransforms/Hough Transform  DialogController=vipDDGCreate  DialogControllerArgs=DataTag12  theta_res=pi/180  rho_res=1  out_theta_rho=on  outdtmode=double  firstCoeffMode=Binary point scaling  firstCoeffWordLength=16  firstCoeffFracLength=14  secondCoeffMode=Binary point scaling  secondCoeffWordLength=32  secondCoeffFracLength=16  outputMode=Binary point scaling  outputWordLength=16  outputFracLength=0  accumMode=Binary point scaling  accumWordLength=32  accumFracLength=20  prodOutputMode=Binary point scaling  prodOutputWordLength=32  prodOutputFracLength=20  memoryMode=Binary point scaling  memoryWordLength=32  memoryFracLength=16  roundingMode=Nearest  overflowMode=on
  Identify Validation Gate : Stateflow chart  TreatAsAtomicUnit=on
  If Action Subsystem : Subsystem  TreatAsAtomicUnit=on
  If1 : If  ShowElse=off
  which_camera : Constant  Value=0  SampleTime=-1
  R_forward_out : Outport  OutDataTypeStr=double
  G_forward_out : Outport  Port=2  OutDataTypeStr=double
  B_forward_out : Outport  Port=3  OutDataTypeStr=double
  TargetSelect : Outport  Port=4  OutDataTypeStr=double
  MaintainHeading : Outport  Port=5  OutDataTypeStr=double
  TargetY : Outport  Port=6  OutDataTypeStr=double
  TargetZ : Outport  Port=7  OutDataTypeStr=double
  TargetYaw : Outport  Port=8  OutDataTypeStr=double
  TargetDetected : Outport  Port=9  OutDataTypeStr=double
  wires:
  Constant1/1 -> Identify Validation Gate/4(target_height)
  Constant2/1 -> Identify Validation Gate/5(gate_aspect_ratio)
  Forward_Camera_Dimensions/1 -> Identify Validation Gate/6(Forward_Camera_Dimensions)
  Forward_Fov/1 -> Identify Validation Gate/7(Forward_Fov)
  Identify Validation Gate/1(target_y) -> If Action Subsystem/6(y_in), TargetY/1
  Identify Validation Gate/2(target_z) -> If Action Subsystem/7(z_in), TargetZ/1
  If1/1 -> If Action Subsystem/Action
  which_camera/1 -> If Action Subsystem/4(which_camera)
  output_image/1 -> If1/1
  bw_image/1 -> Edge Detection/1
  Forward_Camera_Dimensions1/1 -> If Action Subsystem/8(Camera_Dimensions)
  Hough Transform1/1 -> Identify Validation Gate/1(hough_table)
  Hough Transform1/2 -> Identify Validation Gate/2(theta_in)
  Hough Transform1/3 -> Identify Validation Gate/3(rho_in)
  Edge Detection/1 -> Hough Transform1/1
  If Action Subsystem/1(R_out) -> R_forward_out/1
  If Action Subsystem/2(G_out) -> G_forward_out/1
  If Action Subsystem/3(B_out) -> B_forward_out/1
  Constant3/1 -> TargetSelect/1
  Constant4/1 -> MaintainHeading/1
  Identify Validation Gate/3(target_yaw) -> TargetYaw/1
  Identify Validation Gate/4(gate_found) -> TargetDetected/1
  R_in/1 -> If Action Subsystem/1(R_in)
  G_in/1 -> If Action Subsystem/2(G_in)
  B_in/1 -> If Action Subsystem/3(B_in)

== system VisionModel_v8/Blob_Analysis/IterativeSegmentation ==
  R : Inport
  G : Inport  Port=2
  B : Inport  Port=3
  Iter_Segment_Thresh : Inport  Port=4
  Color Space  Conversion1 : vipconversions/Color Space  Conversion  conversion=Obsolete  conversionActive=sR'G'B' to L*a*b*  wp_str=D50  rec=Rec. 601 (SDTV)  sys=1125/60/2:1  imagePorts=Separate color signals
  Low Pass Filter : Subsystem
  Segmentation : Subsystem
  LabelMatrix : Outport
  num_colors : Outport  Port=2
  ref_colors : Outport  Port=3
  wires:
  Low Pass Filter/3(B') -> Color Space  Conversion1/3
  Low Pass Filter/2(G') -> Color Space  Conversion1/2
  Low Pass Filter/1(R') -> Color Space  Conversion1/1
  Color Space  Conversion1/3 -> Segmentation/3(b)
  Color Space  Conversion1/2 -> Segmentation/2(a)
  Color Space  Conversion1/1 -> Segmentation/1(L)
  R/1 -> Low Pass Filter/1(R)
  G/1 -> Low Pass Filter/2(G)
  B/1 -> Low Pass Filter/3(B)
  Segmentation/1(LabelMatrix) -> LabelMatrix/1
  Segmentation/2(num_colors) -> num_colors/1
  Segmentation/3(ref_colors) -> ref_colors/1
  Iter_Segment_Thresh/1 -> Segmentation/4(Iter_Segment_Thresh)

== system VisionModel_v8/Blob_Analysis/Segmented Image ==
  LabelMatrix : Inport
  ref_colors : Inport  Port=2
  Action Port : ActionPort  ActionType=then
  Color Space  Conversion : vipconversions/Color Space  Conversion  conversion=Obsolete  conversionActive=L*a*b* to sR'G'B'  wp_str=D65  rec=Rec. 601 (SDTV)  sys=1125/60/2:1  imagePorts=Separate color signals
  Display Image : Stateflow chart  TreatAsAtomicUnit=on
  R_out : Outport
  G_out : Outport  Port=2
  B_out : Outport  Port=3
  wires:
  LabelMatrix/1 -> Display Image/1(LabelMatrix)
  ref_colors/1 -> Display Image/2(ref_colors)
  Display Image/1(L) -> Color Space  Conversion/1
  Display Image/2(a) -> Color Space  Conversion/2
  Display Image/3(b) -> Color Space  Conversion/3
  Color Space  Conversion/1 -> R_out/1
  Color Space  Conversion/2 -> G_out/1
  Color Space  Conversion/3 -> B_out/1

== system VisionModel_v8/Blob_Analysis1/IterativeSegmentation ==
  R : Inport
  G : Inport  Port=2
  B : Inport  Port=3
  Iter_Segment_Thresh : Inport  Port=4
  Color Space  Conversion1 : vipconversions/Color Space  Conversion  conversion=Obsolete  conversionActive=sR'G'B' to L*a*b*  wp_str=D50  rec=Rec. 601 (SDTV)  sys=1125/60/2:1  imagePorts=Separate color signals
  Low Pass Filter : Subsystem
  Segmentation : Subsystem
  LabelMatrix : Outport
  num_colors : Outport  Port=2
  ref_colors : Outport  Port=3
  wires:
  Iter_Segment_Thresh/1 -> Segmentation/4(Iter_Segment_Thresh)
  Segmentation/3(ref_colors) -> ref_colors/1
  Segmentation/2(num_colors) -> num_colors/1
  Segmentation/1(LabelMatrix) -> LabelMatrix/1
  B/1 -> Low Pass Filter/3(B)
  G/1 -> Low Pass Filter/2(G)
  R/1 -> Low Pass Filter/1(R)
  Color Space  Conversion1/1 -> Segmentation/1(L)
  Color Space  Conversion1/2 -> Segmentation/2(a)
  Color Space  Conversion1/3 -> Segmentation/3(b)
  Low Pass Filter/1(R') -> Color Space  Conversion1/1
  Low Pass Filter/2(G') -> Color Space  Conversion1/2
  Low Pass Filter/3(B') -> Color Space  Conversion1/3

== system VisionModel_v8/Blob_Analysis1/Segmented Image ==
  LabelMatrix : Inport
  ref_colors : Inport  Port=2
  Action Port : ActionPort  ActionType=then
  Color Space  Conversion : vipconversions/Color Space  Conversion  conversion=Obsolete  conversionActive=L*a*b* to sR'G'B'  wp_str=D65  rec=Rec. 601 (SDTV)  sys=1125/60/2:1  imagePorts=Separate color signals
  Display Image : Stateflow chart  TreatAsAtomicUnit=on
  R_out : Outport
  G_out : Outport  Port=2
  B_out : Outport  Port=3
  wires:
  Color Space  Conversion/3 -> B_out/1
  Color Space  Conversion/2 -> G_out/1
  Color Space  Conversion/1 -> R_out/1
  Display Image/3(b) -> Color Space  Conversion/3
  Display Image/2(a) -> Color Space  Conversion/2
  Display Image/1(L) -> Color Space  Conversion/1
  ref_colors/1 -> Display Image/2(ref_colors)
  LabelMatrix/1 -> Display Image/1(LabelMatrix)

== system VisionModel_v8/ColorSelect/L_detector ==
  Action Port : ActionPort  ActionType=elseif
  ColorFilter1 : Constant  Value=[0 0 0 0 0 0 1]  SampleTime=-1
  OutputSegmentedImage1 : Constant  Value=0  SampleTime=-1
  ColorFilter : Outport  OutDataTypeStr=double
  OutputSegmentedImage : Outport  Port=2  OutDataTypeStr=double
  wires:
  ColorFilter1/1 -> ColorFilter/1
  OutputSegmentedImage1/1 -> OutputSegmentedImage/1

== system VisionModel_v8/ColorSelect/buoy_detector ==
  Action Port : ActionPort  ActionType=elseif
  ColorFilter1 : Constant  Value=[0 0 1 1 1 1 1]  SampleTime=-1
  OutputSegmentedImage1 : Constant  SampleTime=-1
  ColorFilter : Outport  OutDataTypeStr=double
  OutputSegmentedImage : Outport  Port=2  OutDataTypeStr=double
  wires:
  ColorFilter1/1 -> ColorFilter/1
  OutputSegmentedImage1/1 -> OutputSegmentedImage/1

== system VisionModel_v8/ColorSelect/drop_mech ==
  Action Port : ActionPort  ActionType=elseif
  ColorFilter1 : Constant  Value=[1 1 0 1 0 0 0]  SampleTime=-1
  OutputSegmentedImage1 : Constant  Value=0  SampleTime=-1
  ColorFilter : Outport  OutDataTypeStr=double
  OutputSegmentedImage : Outport  Port=2  OutDataTypeStr=double
  wires:
  OutputSegmentedImage1/1 -> OutputSegmentedImage/1
  ColorFilter1/1 -> ColorFilter/1

== system VisionModel_v8/ColorSelect/path_detector ==
  Action Port : ActionPort  ActionType=elseif
  ColorFilter1 : Constant  Value=[0 0 0 0 1 1 0]  SampleTime=-1
  OutputSegmentedImage1 : Constant  Value=0  SampleTime=-1
  ColorFilter : Outport  OutDataTypeStr=double
  OutputSegmentedImage : Outport  Port=2  OutDataTypeStr=double
  wires:
  OutputSegmentedImage1/1 -> OutputSegmentedImage/1
  ColorFilter1/1 -> ColorFilter/1

== system VisionModel_v8/ColorSelect/torpedo ==
  Action Port : ActionPort  ActionType=elseif
  ColorFilter1 : Constant  Value=[0 0 1 1 0 0 0]  SampleTime=-1
  OutputSegmentedImage1 : Constant  Value=0  SampleTime=-1
  ColorFilter : Outport  OutDataTypeStr=double
  OutputSegmentedImage : Outport  Port=2  OutDataTypeStr=double
  wires:
  OutputSegmentedImage1/1 -> OutputSegmentedImage/1
  ColorFilter1/1 -> ColorFilter/1

== system VisionModel_v8/ColorSelect/validation_gate ==
  Action Port : ActionPort  ActionType=then
  ColorFilter1 : Constant  Value=[1 0 0 0 1 0 0]  SampleTime=-1
  OutputSegmentedImage1 : Constant  SampleTime=-1
  ColorFilter : Outport  OutDataTypeStr=double
  OutputSegmentedImage : Outport  Port=2  OutDataTypeStr=double
  wires:
  ColorFilter1/1 -> ColorFilter/1
  OutputSegmentedImage1/1 -> OutputSegmentedImage/1

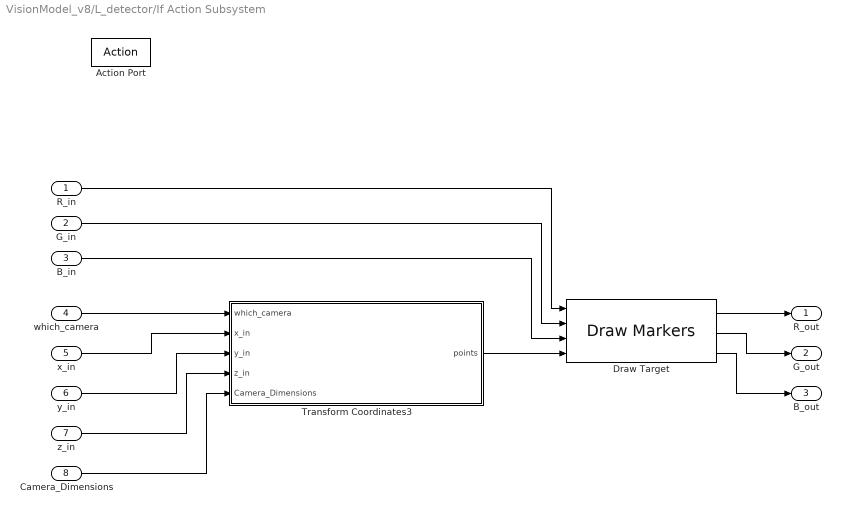
== system VisionModel_v8/L_detector/If Action Subsystem ==
  R_in : Inport
  G_in : Inport  Port=2
  B_in : Inport  Port=3
  which_camera : Inport  Port=4
  x_in : Inport  Port=5
  y_in : Inport  Port=6
  z_in : Inport  Port=7
  Camera_Dimensions : Inport  Port=8
  Action Port : ActionPort  ActionType=then
  Draw Target : viptextngfix/Draw Markers  DialogController=vipDDGCreate  DialogControllerArgs=DataTag8  shape=X-mark  size=7  fill=off  fillClrSource=Specify via dialog  display=User-specified value  intensity=200  color=[1 0 0]  opacity=0.6  viewport=Entire image  antialiasing=off  inType=Obsolete  imagePorts=Separate color signals  prodOutputMode=Binary point scaling  prodOutputWordLength=32  prodOutputFracLength=14  memoryMode=Specify word length  memoryWordLength=16  memoryFracLength=15  roundingMode=Floor  overflowMode=off
  Transform Coordinates3 : Stateflow chart  TreatAsAtomicUnit=on
  R_out : Outport  OutDataTypeStr=double
  G_out : Outport  Port=2  OutDataTypeStr=double
  B_out : Outport  Port=3  OutDataTypeStr=double
  wires:
  which_camera/1 -> Transform Coordinates3/1(which_camera)
  x_in/1 -> Transform Coordinates3/2(x_in)
  y_in/1 -> Transform Coordinates3/3(y_in)
  z_in/1 -> Transform Coordinates3/4(z_in)
  Camera_Dimensions/1 -> Transform Coordinates3/5(Camera_Dimensions)
  Draw Target/1 -> R_out/1
  Transform Coordinates3/1(points) -> Draw Target/4
  Draw Target/2 -> G_out/1
  Draw Target/3 -> B_out/1
  R_in/1 -> Draw Target/1
  G_in/1 -> Draw Target/2
  B_in/1 -> Draw Target/3

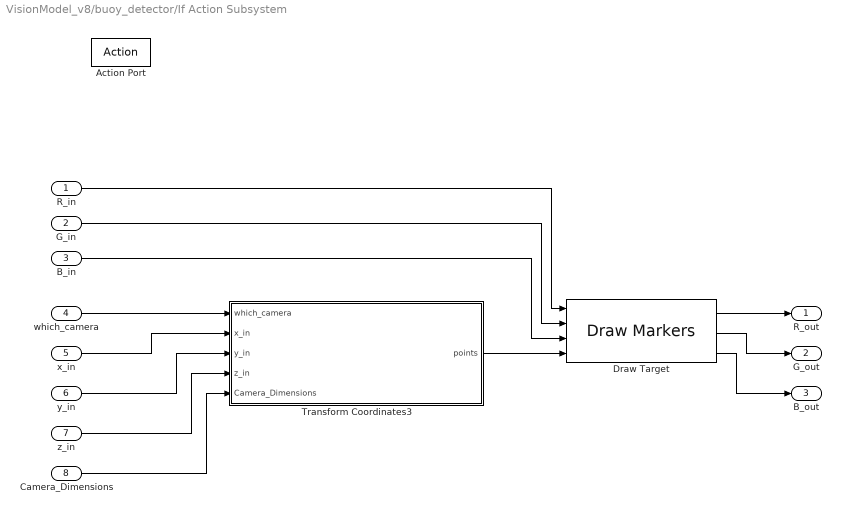
== system VisionModel_v8/buoy_detector/If Action Subsystem ==
  R_in : Inport
  G_in : Inport  Port=2
  B_in : Inport  Port=3
  which_camera : Inport  Port=4
  x_in : Inport  Port=5
  y_in : Inport  Port=6
  z_in : Inport  Port=7
  Camera_Dimensions : Inport  Port=8
  Action Port : ActionPort  ActionType=then
  Draw Target : viptextngfix/Draw Markers  DialogController=vipDDGCreate  DialogControllerArgs=DataTag9  shape=X-mark  size=7  fill=off  fillClrSource=Specify via dialog  display=User-specified value  intensity=200  color=[1 0 0]  opacity=0.6  viewport=Entire image  antialiasing=off  inType=Obsolete  imagePorts=Separate color signals  prodOutputMode=Binary point scaling  prodOutputWordLength=32  prodOutputFracLength=14  memoryMode=Specify word length  memoryWordLength=16  memoryFracLength=15  roundingMode=Floor  overflowMode=off
  Transform Coordinates3 : Stateflow chart  TreatAsAtomicUnit=on
  R_out : Outport  OutDataTypeStr=double
  G_out : Outport  Port=2  OutDataTypeStr=double
  B_out : Outport  Port=3  OutDataTypeStr=double
  wires:
  which_camera/1 -> Transform Coordinates3/1(which_camera)
  x_in/1 -> Transform Coordinates3/2(x_in)
  y_in/1 -> Transform Coordinates3/3(y_in)
  z_in/1 -> Transform Coordinates3/4(z_in)
  Camera_Dimensions/1 -> Transform Coordinates3/5(Camera_Dimensions)
  Draw Target/1 -> R_out/1
  Draw Target/2 -> G_out/1
  Draw Target/3 -> B_out/1
  R_in/1 -> Draw Target/1
  G_in/1 -> Draw Target/2
  B_in/1 -> Draw Target/3
  Transform Coordinates3/1(points) -> Draw Target/4

== system VisionModel_v8/torpedo/If Action Subsystem ==
  R_in : Inport
  G_in : Inport  Port=2
  B_in : Inport  Port=3
  which_camera : Inport  Port=4
  x_in : Inport  Port=5
  y_in : Inport  Port=6
  z_in : Inport  Port=7
  Camera_Dimensions : Inport  Port=8
  Action Port : ActionPort  ActionType=then
  Draw Target : viptextngfix/Draw Markers  DialogController=vipDDGCreate  DialogControllerArgs=DataTag10  shape=X-mark  size=7  fill=off  fillClrSource=Specify via dialog  display=User-specified value  intensity=200  color=[1 0 0]  opacity=0.6  viewport=Entire image  antialiasing=off  inType=Obsolete  imagePorts=Separate color signals  prodOutputMode=Binary point scaling  prodOutputWordLength=32  prodOutputFracLength=14  memoryMode=Specify word length  memoryWordLength=16  memoryFracLength=15  roundingMode=Floor  overflowMode=off
  Transform Coordinates3 : Stateflow chart  TreatAsAtomicUnit=on
  R_out : Outport  OutDataTypeStr=double
  G_out : Outport  Port=2  OutDataTypeStr=double
  B_out : Outport  Port=3  OutDataTypeStr=double
  wires:
  which_camera/1 -> Transform Coordinates3/1(which_camera)
  x_in/1 -> Transform Coordinates3/2(x_in)
  y_in/1 -> Transform Coordinates3/3(y_in)
  z_in/1 -> Transform Coordinates3/4(z_in)
  Camera_Dimensions/1 -> Transform Coordinates3/5(Camera_Dimensions)
  Draw Target/1 -> R_out/1
  Transform Coordinates3/1(points) -> Draw Target/4
  Draw Target/2 -> G_out/1
  Draw Target/3 -> B_out/1
  R_in/1 -> Draw Target/1
  G_in/1 -> Draw Target/2
  B_in/1 -> Draw Target/3
